simulink model "Task17"  (R2019b)
settings: Solver=VariableStepAuto  StartTime=0.0  StopTime=10  RelTol=1e-3
values from neighbouring files (symbols this model uses):
  A1 = 0.123    [Task17_main.m]
  A2 = 0.0411    [Task17_main.m]
  Cd1 = 0.1    [Task17_main.m]
  Cd2 = 0.4    [Task17_main.m]
  g = 9.81    [Task17_main.m]
  m = 1    [Task17_main.m]
  rho = 1.225    [Task17_main.m]
settings Model: Creator=12393  LastModifiedBy=12393

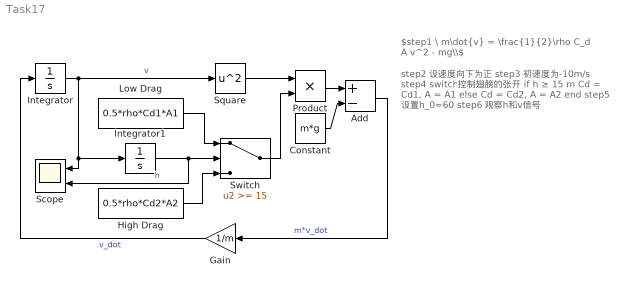
== system Task17 ==
  note: step2 设速度向下为正
      | step3 初速度为-10m/s
      | step4 switch控制翅膀的张开
      | if h ≥ 15 m
      | Cd = Cd1, A = A1
      | else
      | Cd = Cd2, A = A2
      | end
      | step5 设置h_0=60
      | step6 观察h和v信号
  note: $step1 \ m\dot{v} = \frac{1}{2}\rho C_d A v^2 - mg\\$
  Add : Sum  Inputs=+-
  Constant : Constant  Value=m*g
  Gain : Gain  Gain=1/m
  High Drag : Constant  Value=0.5*rho*Cd2*A2
  Integrator : Integrator  InitialCondition=-10
  Integrator1 : Integrator  InitialCondition=60
  Low Drag : Constant  Value=0.5*rho*Cd1*A1
  Product : Product
  Scope : Scope  NumInputPorts=2
  Square : Math  Operator=square  SignedPower=off  SaturateOnIntegerOverflow=on
  Switch : Switch  Threshold=15
  wires:
  Add/1 -> Gain/1  "m*v_dot"
  Switch/1 -> Product/2
  Integrator1/1 -> Scope/2, Switch/2  "h"
  Constant/1 -> Add/2
  High Drag/1 -> Switch/3
  Low Drag/1 -> Switch/1
  Integrator/1 -> Scope/1, Integrator1/1, Square/1  "v"
  Square/1 -> Product/1
  Product/1 -> Add/1
  Gain/1 -> Integrator/1  "v_dot"
